simulink model "pmpc_hil"  (R2024b)
settings: Solver=ode1  StartTime=0  StopTime=10  FixedStep=0.001  RelTol=1e-3
libraries: simulink x1
settings Model: Creator=user  LastModifiedBy=user
settings OptimizationCC: ZeroExternalMemoryAtStartup=off  ZeroInternalMemoryAtStartup=off
settings RTWCC: TargetLang=C++
settings GRTTargetCC: TargetLangStandard=C++11 (ISO)  CodeInterfacePackaging=C++ class

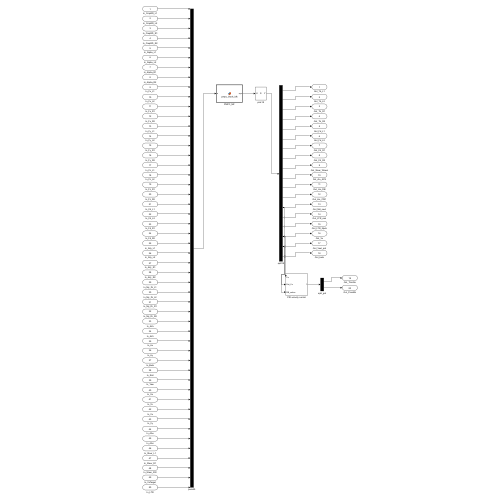
[thumbnail: Simulink's stored preview of the top-level diagram]
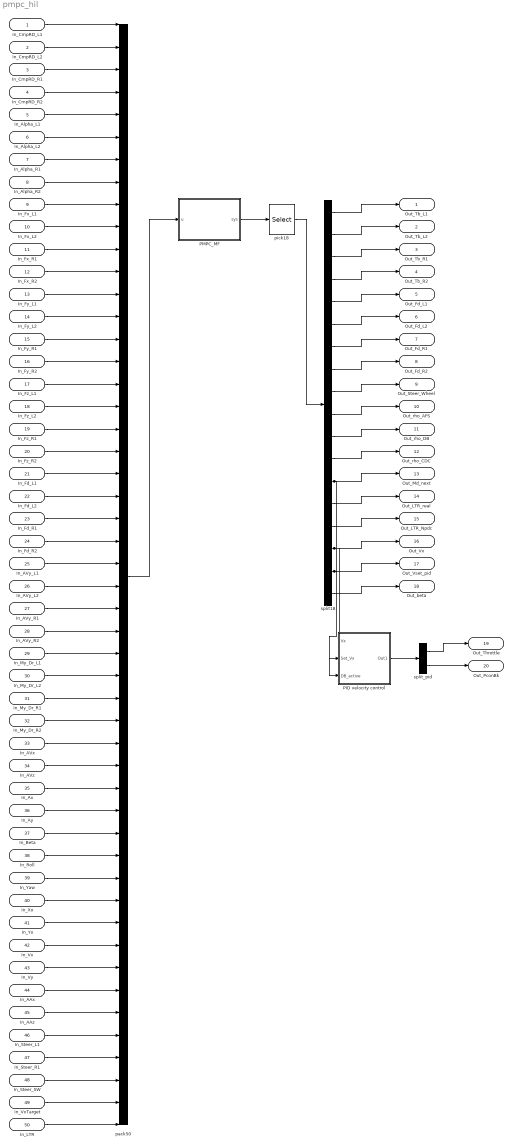
== system pmpc_hil ==
  In_CmpRD_L1 : Inport
  In_CmpRD_L2 : Inport  Port=2
  In_CmpRD_R1 : Inport  Port=3
  In_CmpRD_R2 : Inport  Port=4
  In_Alpha_L1 : Inport  Port=5
  In_Alpha_L2 : Inport  Port=6
  In_Alpha_R1 : Inport  Port=7
  In_Alpha_R2 : Inport  Port=8
  In_Fx_L1 : Inport  Port=9
  In_Fx_L2 : Inport  Port=10
  In_Fx_R1 : Inport  Port=11
  In_Fx_R2 : Inport  Port=12
  In_Fy_L1 : Inport  Port=13
  In_Fy_L2 : Inport  Port=14
  In_Fy_R1 : Inport  Port=15
  In_Fy_R2 : Inport  Port=16
  In_Fz_L1 : Inport  Port=17
  In_Fz_L2 : Inport  Port=18
  In_Fz_R1 : Inport  Port=19
  In_Fz_R2 : Inport  Port=20
  In_Fd_L1 : Inport  Port=21
  In_Fd_L2 : Inport  Port=22
  In_Fd_R1 : Inport  Port=23
  In_Fd_R2 : Inport  Port=24
  In_AVy_L1 : Inport  Port=25
  In_AVy_L2 : Inport  Port=26
  In_AVy_R1 : Inport  Port=27
  In_AVy_R2 : Inport  Port=28
  In_My_Dr_L1 : Inport  Port=29
  In_My_Dr_L2 : Inport  Port=30
  In_My_Dr_R1 : Inport  Port=31
  In_My_Dr_R2 : Inport  Port=32
  In_AVx : Inport  Port=33
  In_AVz : Inport  Port=34
  In_Ax : Inport  Port=35
  In_Ay : Inport  Port=36
  In_Beta : Inport  Port=37
  In_Roll : Inport  Port=38
  In_Yaw : Inport  Port=39
  In_Xo : Inport  Port=40
  In_Yo : Inport  Port=41
  In_Vx : Inport  Port=42
  In_Vy : Inport  Port=43
  In_AAx : Inport  Port=44
  In_AAz : Inport  Port=45
  In_Steer_L1 : Inport  Port=46
  In_Steer_R1 : Inport  Port=47
  In_Steer_SW : Inport  Port=48
  In_VxTarget : Inport  Port=49
  In_LTR : Inport  Port=50
  PID velocity control : Subsystem
  PMPC_MF : MATLAB Function  TreatAsAtomicUnit=on
  pack50 : Mux  Inputs=50
  pick18 : Selector  InputPortWidth=54  IndexOptions=Index vector (dialog)  Indices=[1 2 3 4 5 6 7 8 9 14 15 16 21 29 30 31 32 38]  OutputSizes=1
  split18 : Demux  Outputs=18
  split_pid : Demux  Outputs=2
  Out_Tb_L1 : Outport
  Out_Tb_L2 : Outport  Port=2
  Out_Tb_R1 : Outport  Port=3
  Out_Tb_R2 : Outport  Port=4
  Out_Fd_L1 : Outport  Port=5
  Out_Fd_L2 : Outport  Port=6
  Out_Fd_R1 : Outport  Port=7
  Out_Fd_R2 : Outport  Port=8
  Out_Steer_Wheel : Outport  Port=9
  Out_rho_AFS : Outport  Port=10
  Out_rho_DB : Outport  Port=11
  Out_rho_CDC : Outport  Port=12
  Out_Md_next : Outport  Port=13
  Out_LTR_real : Outport  Port=14
  Out_LTR_Npdc : Outport  Port=15
  Out_Vx : Outport  Port=16
  Out_Vset_pid : Outport  Port=17
  Out_beta : Outport  Port=18
  Out_Throttle : Outport  Port=19
  Out_PconBk : Outport  Port=20
  wires:
  In_CmpRD_L1/1 -> pack50/1
  In_CmpRD_L2/1 -> pack50/2
  In_CmpRD_R1/1 -> pack50/3
  In_CmpRD_R2/1 -> pack50/4
  In_Alpha_L1/1 -> pack50/5
  In_Alpha_L2/1 -> pack50/6
  In_Alpha_R1/1 -> pack50/7
  In_Alpha_R2/1 -> pack50/8
  In_Fx_L1/1 -> pack50/9
  In_Fx_L2/1 -> pack50/10
  In_Fx_R1/1 -> pack50/11
  In_Fx_R2/1 -> pack50/12
  In_Fy_L1/1 -> pack50/13
  In_Fy_L2/1 -> pack50/14
  In_Fy_R1/1 -> pack50/15
  In_Fy_R2/1 -> pack50/16
  In_Fz_L1/1 -> pack50/17
  In_Fz_L2/1 -> pack50/18
  In_Fz_R1/1 -> pack50/19
  In_Fz_R2/1 -> pack50/20
  In_Fd_L1/1 -> pack50/21
  In_Fd_L2/1 -> pack50/22
  In_Fd_R1/1 -> pack50/23
  In_Fd_R2/1 -> pack50/24
  In_AVy_L1/1 -> pack50/25
  In_AVy_L2/1 -> pack50/26
  In_AVy_R1/1 -> pack50/27
  In_AVy_R2/1 -> pack50/28
  In_My_Dr_L1/1 -> pack50/29
  In_My_Dr_L2/1 -> pack50/30
  In_My_Dr_R1/1 -> pack50/31
  In_My_Dr_R2/1 -> pack50/32
  In_AVx/1 -> pack50/33
  In_AVz/1 -> pack50/34
  In_Ax/1 -> pack50/35
  In_Ay/1 -> pack50/36
  In_Beta/1 -> pack50/37
  In_Roll/1 -> pack50/38
  In_Yaw/1 -> pack50/39
  In_Xo/1 -> pack50/40
  In_Yo/1 -> pack50/41
  In_Vx/1 -> pack50/42
  In_Vy/1 -> pack50/43
  In_AAx/1 -> pack50/44
  In_AAz/1 -> pack50/45
  In_Steer_L1/1 -> pack50/46
  In_Steer_R1/1 -> pack50/47
  In_Steer_SW/1 -> pack50/48
  In_VxTarget/1 -> pack50/49
  In_LTR/1 -> pack50/50
  pack50/1 -> PMPC_MF/1(u)
  PMPC_MF/1(sys) -> pick18/1
  pick18/1 -> split18/1
  split18/1 -> Out_Tb_L1/1
  split18/2 -> Out_Tb_L2/1
  split18/3 -> Out_Tb_R1/1
  split18/4 -> Out_Tb_R2/1
  split18/5 -> Out_Fd_L1/1
  split18/6 -> Out_Fd_L2/1
  split18/7 -> Out_Fd_R1/1
  split18/8 -> Out_Fd_R2/1
  split18/9 -> Out_Steer_Wheel/1
  split18/10 -> Out_rho_AFS/1
  split18/11 -> Out_rho_DB/1
  split18/12 -> Out_rho_CDC/1
  split18/13 -> Out_Md_next/1, PID velocity control/3(DB_active)
  split18/14 -> Out_LTR_real/1
  split18/15 -> Out_LTR_Npdc/1
  split18/16 -> Out_Vx/1, PID velocity control/1(Vx)
  split18/17 -> Out_Vset_pid/1, PID velocity control/2(Set_Vx)
  split18/18 -> Out_beta/1
  PID velocity control/1(Out1) -> split_pid/1
  split_pid/1 -> Out_Throttle/1
  split_pid/2 -> Out_PconBk/1

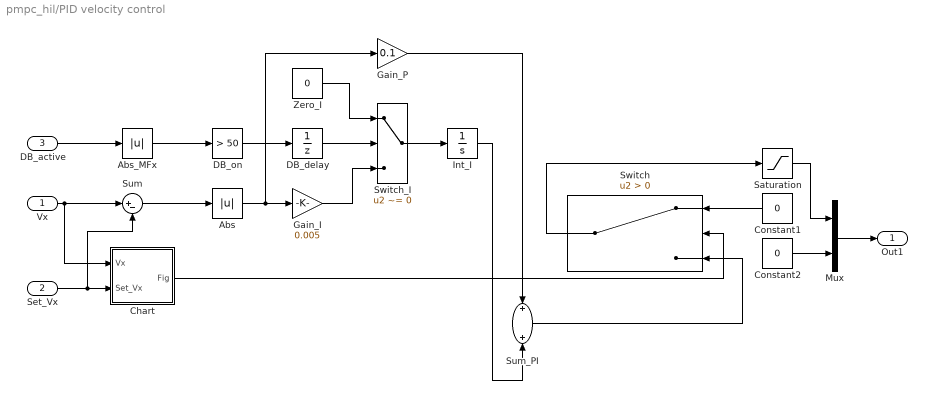
== system pmpc_hil/PID velocity control ==
  Vx : Inport
  Set_Vx : Inport  Port=2
  DB_active : Inport  Port=3
  Abs : Abs  SaturateOnIntegerOverflow=off
  Abs_MFx : Abs  SaturateOnIntegerOverflow=off
  Chart : Stateflow chart  TreatAsAtomicUnit=on
  Constant1 : Constant  Value=0
  Constant2 : Constant  Value=0
  DB_delay : UnitDelay  SampleTime=-1  HasFrameUpgradeWarning=on
  DB_on : simulink/Logic and Bit Operations/Compare To Constant  relop=>  const=50  OutDataTypeStr=uint8
  Gain_I : Gain  Gain=0.005
  Gain_P : Gain  Gain=0.1
  Int_I : Integrator
  Mux : Mux  Inputs=2
  Saturation : Saturate  UpperLimit=1  LowerLimit=0
  Sum : Sum  Inputs=|+-
  Sum_PI : Sum
  Switch : Switch  Criteria=u2 > Threshold  SaturateOnIntegerOverflow=off  InputSameDT=off
  Switch_I : Switch  Criteria=u2 ~= 0  SaturateOnIntegerOverflow=off  InputSameDT=off
  Zero_I : Constant  Value=0
  Out1 : Outport
  wires:
  Mux/1 -> Out1/1
  Constant2/1 -> Mux/2
  Switch/1 -> Saturation/1
  Sum_PI/1 -> Switch/3
  Int_I/1 -> Sum_PI/2
  Switch_I/1 -> Int_I/1
  Gain_P/1 -> Sum_PI/1
  Constant1/1 -> Switch/1
  Gain_I/1 -> Switch_I/3
  Zero_I/1 -> Switch_I/1
  Abs/1 -> Gain_I/1, Gain_P/1
  Sum/1 -> Abs/1
  Saturation/1 -> Mux/1
  Abs_MFx/1 -> DB_on/1
  DB_on/1 -> DB_delay/1
  Vx/1 -> Sum/1, Chart/1(Vx)
  DB_delay/1 -> Switch_I/2
  DB_active/1 -> Abs_MFx/1
  Set_Vx/1 -> Chart/2(Set_Vx), Sum/2
  Chart/1(Fig) -> Switch/2

== matlab function pmpc_hil/PMPC_MF ==
  settings: updateMethod=DISCRETE  sampleTime=0.01
  data: u input; sys output; PMPC_P parameter
function sys = pmpc_block_blk(u, PMPC_P)
%#codegen
%  块里只写一行调用 —— 实体在 pmpc_block.m,
%  这样可以单独对它跑 codegen 调试(见 cg_block.m)。
sys = pmpc_block(u, PMPC_P);
end

== stateflow chart pmpc_hil/PID velocity control/Chart ==
  (default) -> (junction 4)
  (junction 4) -> (junction 7) [order 2] : [Vx>=Set_Vx]
  (junction 4) -> (junction 6) [order 1] : [Vx<Set_Vx]{Fig=-1;}
  (junction 7) -> (junction 11)
  (junction 11) -> (junction 13) [order 1] : [Vx>Set_Vx]{Fig=1;}
  (junction 11) -> (junction 15) [order 2] : [Vx==Set_Vx]{Fig=0;}
  (junction 13) -> (junction 17)
  (junction 15) -> (junction 6)
  (junction 17) -> (junction 15)
  data: Vx input double; Set_Vx input double; Fig output
